simulink model "manipulator"  (R2018a)
settings: Solver=FixedStepAuto  StartTime=0.0  StopTime=100.0  FixedStep=0.01  RelTol=1e-3
settings Model: Creator=Петр  LastModifiedBy=Петр

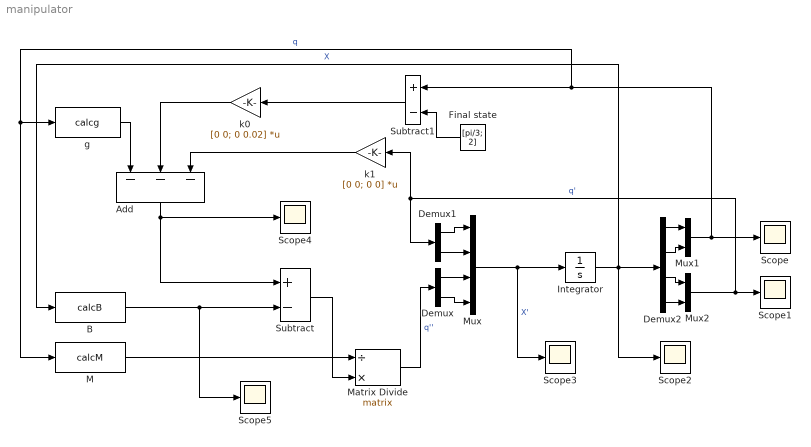
== system manipulator ==
  Add : Sum  Inputs=---
  B : MATLABFcn  MATLABFcn=calcB  OutputDimensions=[2 1]  Output1D=off
  Demux : Demux  Outputs=2
  Demux1 : Demux  Outputs=2
  Demux2 : Demux
  Final state : Constant  Value=[pi/3; 2]
  Integrator : Integrator  InitialCondition=[0; 0; 0; 0]  UpperSaturationLimit=10000  LowerSaturationLimit=-10000
  M : MATLABFcn  MATLABFcn=calcM  OutputDimensions=[2 2]  Output1D=off
  Matrix Divide : Product  Inputs=/*  Multiplication=Matrix(*)
  Mux : Mux
  Mux1 : Mux  Inputs=2
  Mux2 : Mux  Inputs=2
  Scope{,1..5} (6 alike) : Scope
  Subtract : Sum  Inputs=+-
  Subtract1 : Sum  Inputs=+-
  g : MATLABFcn  MATLABFcn=calcg  OutputDimensions=2
  k0 : Gain  Gain=[0 0; 0 0.02]  Multiplication=Matrix(K*u)
  k1 : Gain  Gain=[0 0; 0 0]  Multiplication=Matrix(K*u)
  wires:
  M/1 -> Matrix Divide/1
  Matrix Divide/1 -> Demux/1  "q''"
  Demux1/1 -> Mux/1
  Demux1/2 -> Mux/2
  Demux/1 -> Mux/3
  Demux/2 -> Mux/4
  Mux/1 -> Scope3/1, Integrator/1  "X'"
  Integrator/1 -> B/1, Scope2/1, Demux2/1  "X"
  Demux2/1 -> Mux1/1
  Demux2/2 -> Mux1/2
  Demux2/4 -> Mux2/2
  Demux2/3 -> Mux2/1
  Mux1/1 -> Scope/1, M/1, g/1, Subtract1/1  "q"
  Mux2/1 -> k1/1, Demux1/1, Scope1/1  "q'"
  Subtract/1 -> Matrix Divide/2
  Final state/1 -> Subtract1/2
  Subtract1/1 -> k0/1
  g/1 -> Add/1
  k0/1 -> Add/2
  k1/1 -> Add/3
  Add/1 -> Subtract/1, Scope4/1
  B/1 -> Subtract/2, Scope5/1
